simulink model "Nodos_primer_control_continua"  (R2019a)
settings: Solver=VariableStepAuto  StartTime=0.0  StopTime=50  RelTol=1e-3
values from neighbouring files (symbols this model uses):
  h = 1.0000e+00    (= 1)    [programa_nodos.m]
undefined symbols (not defined in the file or in its folder): A1, B1, C1
settings Model: Creator=Alejoxbg  LastModifiedBy=Alejoxbg

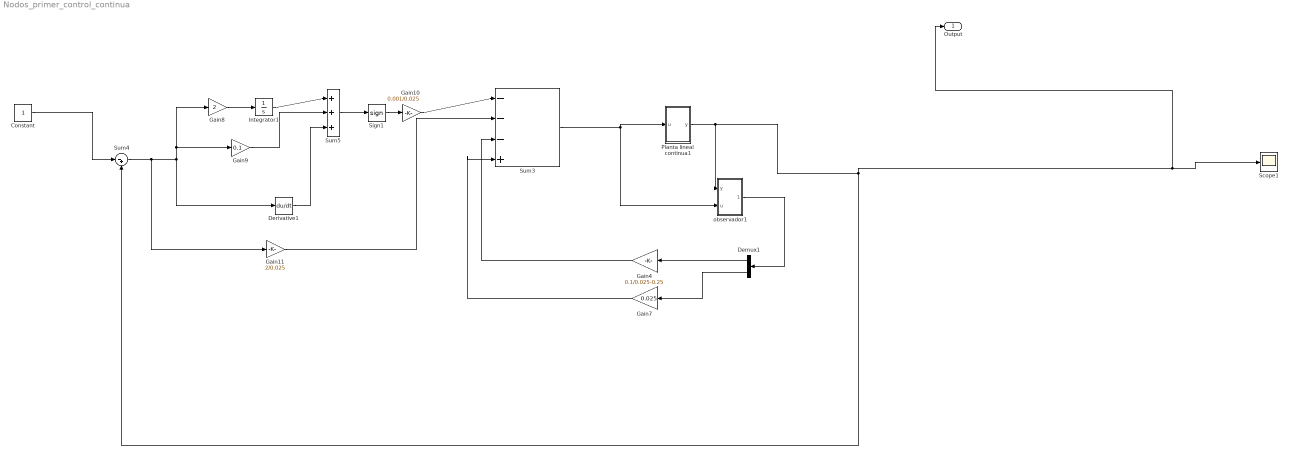
== system Nodos_primer_control_continua ==
  Constant : Constant
  Demux1 : Demux  Outputs=2
  Derivative1 : Derivative
  Gain10 : Gain  Gain=0.001/0.025
  Gain11 : Gain  Gain=2/0.025
  Gain4 : Gain  Gain=0.1/0.025-0.25
  Gain7 : Gain  Gain=0.025
  Gain8 : Gain  Gain=2
  Gain9 : Gain  Gain=0.1
  Integrator1 : Integrator
  Planta lineal continua1 : Subsystem
  Scope1 : Scope
  Sign1 : Signum  ZeroCross=off
  Sum3 : Sum  Inputs=|---+
  Sum4 : Sum  Inputs=|-+
  Sum5 : Sum  Inputs=|+++
  observador1 : Subsystem
  Output : Outport
  wires:
  Gain11/1 -> Sum3/2
  Gain8/1 -> Integrator1/1
  Gain7/1 -> Sum3/4
  Gain4/1 -> Sum3/3
  Sum5/1 -> Sign1/1
  Demux1/2 -> Gain7/1
  Gain9/1 -> Sum5/2
  Sum3/1 -> observador1/2(u), Planta lineal continua1/1(u)
  Integrator1/1 -> Sum5/1
  Derivative1/1 -> Sum5/3
  observador1/1(xgorro) -> Demux1/1
  Sum4/1 -> Gain11/1, Derivative1/1, Gain8/1, Gain9/1
  Demux1/1 -> Gain4/1
  Gain10/1 -> Sum3/1
  Sign1/1 -> Gain10/1
  Planta lineal continua1/1(y) -> observador1/1(y), Output/1, Scope1/1, Sum4/2
  Constant/1 -> Sum4/1

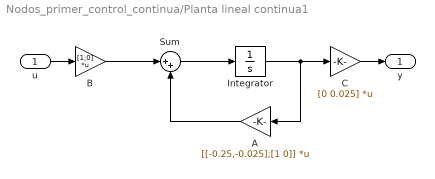
== system Nodos_primer_control_continua/Planta lineal continua1 ==
  u : Inport
  A : Gain  Gain=[[-0.25,-0.025];[1 0]]  Multiplication=Matrix(K*u) (u vector)
  B : Gain  Gain=[1;0]  Multiplication=Matrix(K*u) (u vector)
  C : Gain  Gain=[0 0.025]  Multiplication=Matrix(K*u) (u vector)
  Integrator : Integrator
  Sum : Sum  Inputs=|++
  y : Outport
  wires:
  C/1 -> y/1
  u/1 -> B/1
  Integrator/1 -> A/1, C/1
  A/1 -> Sum/2
  Sum/1 -> Integrator/1
  B/1 -> Sum/1

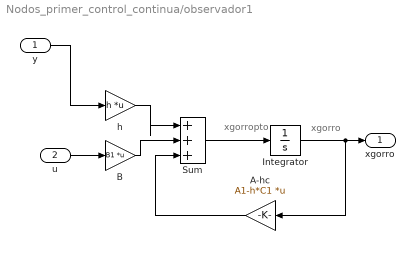
== system Nodos_primer_control_continua/observador1 ==
  note: xgorro
  note: xgorropto
  y : Inport
  u : Inport  Port=2
  A-hc : Gain  Gain=A1-h*C1  Multiplication=Matrix(K*u) (u vector)
  B : Gain  Gain=B1  Multiplication=Matrix(K*u) (u vector)
  Integrator : Integrator
  Sum : Sum  Inputs=|+++
  h : Gain  Gain=h  Multiplication=Matrix(K*u) (u vector)
  xgorro : Outport
  wires:
  u/1 -> B/1
  h/1 -> Sum/1
  B/1 -> Sum/2
  A-hc/1 -> Sum/3
  Integrator/1 -> xgorro/1, A-hc/1
  Sum/1 -> Integrator/1
  y/1 -> h/1
